simulink model "receiveDSBLC_RTLSDR"  (R2017a)
settings: Solver=VariableStepAuto  StartTime=0.0  StopTime=inf  RelTol=1e-3
undefined symbols (not defined in the file or in its folder): designMultirateFIR
libraries: dspsnks4 x1, dspsigops x1, dsparch4 x1, dspmlti4 x1, sdrrlib x1, simulink x1
settings Model: Creator=prust  LastModifiedBy=prust

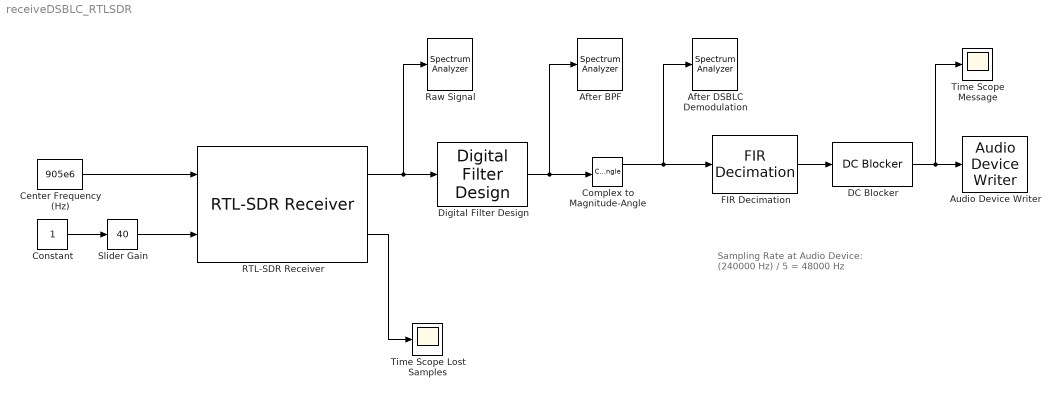
== system receiveDSBLC_RTLSDR ==
  note: Sampling Rate at Audio Device: (240000 Hz) / 5 = 48000 Hz
  After BPF : SpectrumAnalyzer
  After DSBLC Demodulation : SpectrumAnalyzer
  Audio Device Writer : dspsnks4/Audio Device Writer  Driver=DirectSound  Device=Default  InheritSampleRate=on  SampleRate=44100  BitDepth=16-bit integer  BufferSize=4096  NumBuffers=10  DefaultOutputChannelMapping=on  OutputChannelMapping=1:2  OutputNumUnderrunSamples=off  DriverIdx=1  DeviceWarnFlag=''
  Center Frequency (Hz) : Constant  Value=905e6
  Complex to Magnitude-Angle : ComplexToMagnitudeAngle
  Constant : Constant
  DC Blocker : dspsigops/DC Blocker  Algorithm=IIR  NormalizedBandwidth=0.001  Length=8  Order=6  SimulateUsing=Code generation
      settings: SourceProductName=DSP System Toolbox  SourceProductBaseCode=DS
  Digital Filter Design : dsparch4/Digital Filter Design  mwdsp_browser_bugfix_var=off
  FIR Decimation : dspmlti4/FIR Decimation  FilterSource=Auto  h=designMultirateFIR(1,2)  D=5  filtStruct=Direct form  FilterObject=FDECIM  InputProcessing=Columns as channels (frame based)  framing=Enforce single-rate processing  inputOffset=0  outputBufInitCond=0  roundingMode=Floor  overflowMode=off  firstCoeffDataTypeStr=Inherit: Same word length as input  firstCoeffMin=[]  firstCoeffMax=[]  firstCoeffLastDataTypeStr=Inherit: Same word length as input  outputDataTypeStr=Inherit: Same as accumulator  outputMin=[]  outputMax=[]  outputLastDataTypeStr=Inherit: Same as accumulator
  RTL-SDR Receiver : sdrrlib/RTL-SDR Receiver  SourceLibraryInfo="This block requires <a href=\"http://www.mathworks.com/hardware-support/rtl-sdr.html\">Communications System Toolbox Support Package for RTL-SDR Radio</a>"  sobjType=sdrr.internal.SDRRTLReceiverSL  IPAddress=0  dataUDPPort=-1  ctrlUDPPort=-1  subDeviceList=nosubdev  sdrBlockType=SDRBlockTypeSLT.SDRRxBlock  requester=UNUSED_BY_SFCN  sdrExecutionMode=SDRExecutionModeSLT.ExecModeHW  LostSamplesOutputPort=on  OutputDataType=single  FrameLength=1000  EnableBurstMode=off  NumFramesInBurst=20  BypassUserLogic=off  DecimatorSelect=DDC decimator  SourceSelect=RF data  SineAmplitude=16000  EnableInternalClock=off  BypassIQBalance=off  CenterFrequency=102.5e6  IFBandwidth=40e6  ADCRateSource=Dialog  ADCRate=240000  CenterFrequencySource=Input port  GainSource=Input port  IntermediateFrequency=0  Gain=30  DecimationFactorSource=Dialog  DecimationFactor=512  RFFrequencyIsTunable=logical(1)  SampleTime=(1000)/(240000)  IFBandwidthSource=Dialog  SineFrequency=30000  BypassDCBlockingFilter=off  IntermediateFrequencySource=Dialog  IQBalanceCoefficients=64  SkipAllHardwareResetAndInitialization=off  EnableIQCalibrationTable=on  CacheIQCalibrationTable=off  EnableOffsetTuning=off  EnableRTLAGC=off  EnableTestMode=off  EnableTunerAGC=off  FrequencyCorrectionSource=Dialog  FrequencyCorrection=0  NumMLBuffers=128  NumUSBBuffers=16  LatencyOutputPort=off  RTLCrystalFrequency=28800000  TunerCrystalFrequency=28800000
      settings: SourceProductName=Communications System Toolbox Support Package for RTL-SDR Radio  SourceProductBaseCode=RTLSDR
  Raw Signal : SpectrumAnalyzer
  Slider Gain : simulink/Math Operations/Slider Gain  gain=40  low=0  high=60
  Time Scope Lost Samples : Scope
  Time Scope Message : Scope
  wires:
  RTL-SDR Receiver/1 -> Digital Filter Design/1, Raw Signal/1
  Center Frequency (Hz)/1 -> RTL-SDR Receiver/1
  Constant/1 -> Slider Gain/1
  Digital Filter Design/1 -> After BPF/1, Complex to Magnitude-Angle/1
  RTL-SDR Receiver/2 -> Time Scope Lost Samples/1
  Complex to Magnitude-Angle/1 -> FIR Decimation/1, After DSBLC Demodulation/1
  DC Blocker/1 -> Audio Device Writer/1, Time Scope Message/1
  Slider Gain/1 -> RTL-SDR Receiver/2
  FIR Decimation/1 -> DC Blocker/1
